simulink model "model3"  (Simulink 7.1)
settings: Solver=ode45  StartTime=0.0  StopTime=0.5  RelTol=1e-3
undefined symbols (not defined in the file): x
libraries: fuzblock x1
settings Model: Creator=ruchishya  LastModifiedBy=ruchishya
settings DataIOCC: SaveState=on  StateSaveName=x  TimeSaveName=t  OutputSaveName=y

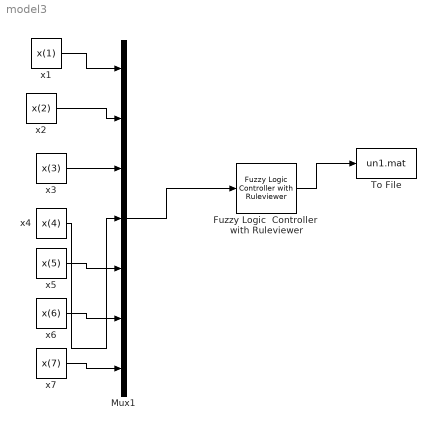
== system model3 ==
  Fuzzy Logic  Controller  with Ruleviewer : fuzblock/Fuzzy Logic  Controller  with Ruleviewer  SystemSampleTime=-1  fismatrix=fuzzyruchi9  Ts=2
  Mux1 : Mux  Inputs=7
  To File : ToFile  Filename=un1.mat  MatrixName=f
  x1 : Constant  Value=x(1)  OutDataType=sfix(16)  OutScaling=2^0
  x2 : Constant  Value=x(2)  OutDataType=sfix(16)  OutScaling=2^0  SampleTime=1
  x3 : Constant  Value=x(3)  OutDataType=sfix(16)  OutScaling=2^0
  x4 : Constant  Value=x(4)  OutDataType=sfix(16)  OutScaling=2^0  SampleTime=1
  x5 : Constant  Value=x(5)  OutDataType=sfix(16)  OutScaling=2^0
  x6 : Constant  Value=x(6)  OutDataType=sfix(16)  OutScaling=2^0
  x7 : Constant  Value=x(7)  OutDataType=sfix(16)  OutScaling=2^0
  wires:
  x2/1 -> Mux1/2
  x6/1 -> Mux1/6
  x7/1 -> Mux1/7
  x5/1 -> Mux1/5
  x3/1 -> Mux1/3
  x1/1 -> Mux1/1
  Mux1/1 -> Fuzzy Logic  Controller  with Ruleviewer/1
  x4/1 -> Mux1/4
  Fuzzy Logic  Controller  with Ruleviewer/1 -> To File/1
